simulink model "velo_pi"  (R2020b)
settings: Solver=VariableStepAuto  StartTime=0.0  StopTime=10  RelTol=1e-3
libraries: arduino_io_lib x5
settings Model: Creator=kei55  LastModifiedBy=kei55

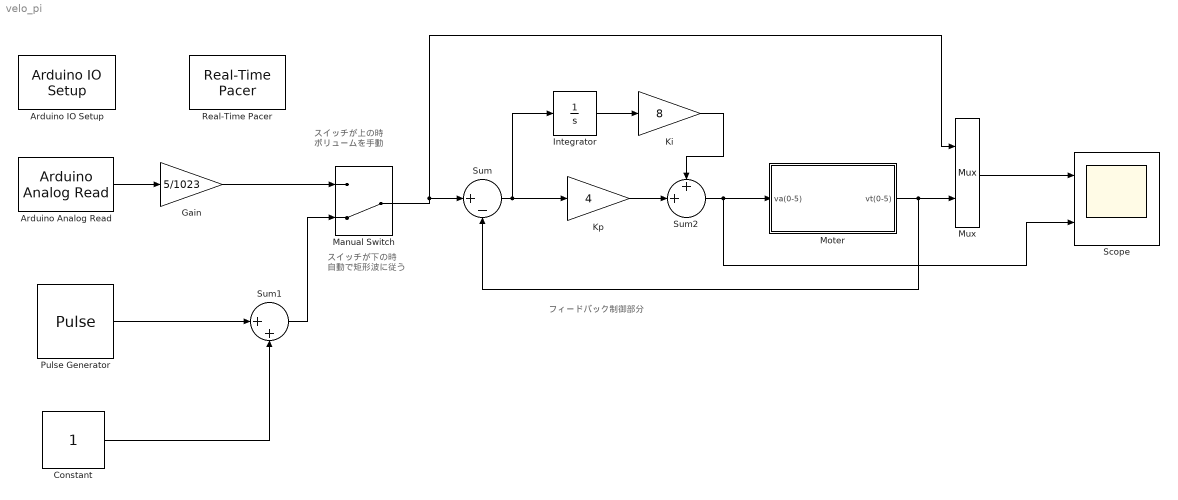
== system velo_pi ==
  note: スイッチが上の時
      | ボリュームを手動
  note: フィードバック制御部分
  note: スイッチが下の時
      | 自動で矩形波に従う
  Arduino Analog Read : arduino_io_lib/Arduino Analog Read  arduinoVar=Temporary arduino variable: Arduino1  arduinoPin=1  T=1/50
  Arduino IO Setup : arduino_io_lib/Arduino IO Setup  Priority=3  arduinoVar=Temporary arduino variable: Arduino1  workspaceVarName=a  comPort=COM3
  Constant : Constant
  Gain : Gain  Gain=5/1023
  Integrator : Integrator
  Ki : Gain  Gain=8
  Kp : Gain  Gain=4
  Manual Switch : ManualSwitch  CurrentSetting=0
  Moter : Subsystem
  Mux : Mux  Inputs=2
  Pulse Generator : DiscretePulseGenerator  PulseType=Time based  Amplitude=0.5  Period=4  PulseWidth=50  SampleTime=1/50
  Real-Time Pacer : arduino_io_lib/Real-Time Pacer  simTimePerRealTime=1
  Scope : Scope  NumInputPorts=2
  Sum : Sum  Inputs=|+-
  Sum1 : Sum  Inputs=|++
  Sum2 : Sum  Inputs=++|
  wires:
  Arduino Analog Read/1 -> Gain/1
  Mux/1 -> Scope/1
  Moter/1(vt(0-5)) -> Sum/2, Mux/2
  Gain/1 -> Manual Switch/1
  Pulse Generator/1 -> Sum1/1
  Constant/1 -> Sum1/2
  Sum1/1 -> Manual Switch/2
  Manual Switch/1 -> Mux/1, Sum/1
  Sum/1 -> Integrator/1, Kp/1
  Sum2/1 -> Scope/2, Moter/1(va(0-5))
  Integrator/1 -> Ki/1
  Ki/1 -> Sum2/1
  Kp/1 -> Sum2/2

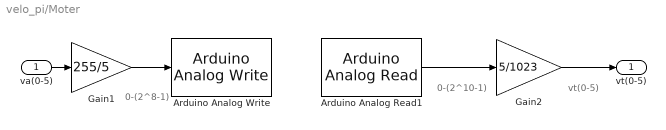
== system velo_pi/Moter ==
  note: 0-(2^8-1)
  note: 0-(2^10-1)
  note: vt(0-5)
  va(0-5) : Inport
  Arduino Analog Read1 : arduino_io_lib/Arduino Analog Read  arduinoVar=Temporary arduino variable: Arduino1  arduinoPin=0  T=1/50
  Arduino Analog Write : arduino_io_lib/Arduino Analog Write  arduinoVar=Temporary arduino variable: Arduino1  arduinoPin=3  T=1/50
  Gain1 : Gain  Gain=255/5
  Gain2 : Gain  Gain=5/1023
  vt(0-5) : Outport
  wires:
  Arduino Analog Read1/1 -> Gain2/1
  Gain1/1 -> Arduino Analog Write/1
  Gain2/1 -> vt(0-5)/1
  va(0-5)/1 -> Gain1/1
